simulink model "verify_ground_storage_U_tube_mdl"  (R2016b)
settings: Solver=ode45  StartTime=0  StopTime=2*3600  MaxStep=100  RelTol=1e-3  EnableMultiTasking=on
libraries: carnot x3, simulink x1
settings Model: Creator=drhf  LastModifiedBy=User
settings DataIOCC: SaveFormat=Array  SignalLoggingSaveFormat=ModelDataLogs
settings OptimizationCC: ExpressionDepthLimit=2147483647  LifeSpan=inf
settings DebuggingCC: UnderspecifiedInitializationDetection=Classic  MergeDetectMultiDrivingBlocksExec=none  SolverPrmCheckMsg=warning  FcnCallInpInsideContextMsg=warning  StateNameClashWarn=warning  SFUnexpectedBacktrackingDiag=warning  SFNoUnconditionalDefaultTransitionDiag=warning  SFExecutionAtInitializationDiag=none
settings HardwareCC: ProdBitPerPointer=32  ProdBitPerSizeT=32  ProdBitPerPtrDiffT=32  ProdLargestAtomicFloat=None  ProdIntDivRoundTo=Undefined  ProdEndianess=Unspecified  ProdWordSize=32  ProdHWDeviceType=32-bit Generic
settings ModelReferenceCC: PropagateSignalLabelsOutOfModel=off
settings GRTTargetCC: TargetLangStandard=C89/C90 (ANSI)  GeneratePreprocessorConditionals=Disable all  CombineOutputUpdateFcns=off  GRTInterface=on
settings ConfigComp: CovMetricSettings=dw  CovHtmlReporting=on  CovSaveCumulativeToWorkspaceVar=on  CovSaveSingleToWorkspaceVar=on  CovExternalEMLEnable=off

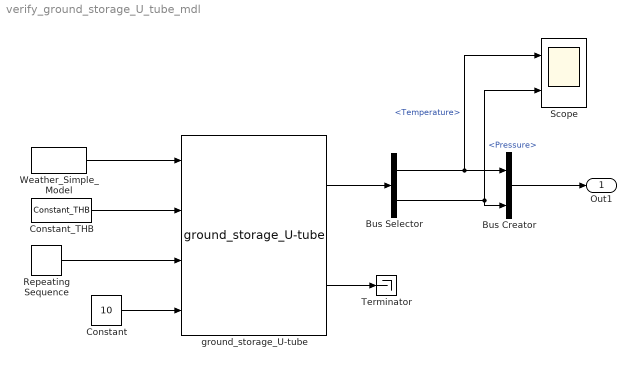
== system verify_ground_storage_U_tube_mdl ==
  Bus Creator : BusCreator  Inputs=2
  Bus Selector : BusSelector  OutputSignals=Temperature,Pressure
  Constant : Constant  Value=10
  Constant_THB : carnot/Source/Simple/Constant_THB  t=40  mdot=600/3600  p=1e5  mID=No Pressure Drop  fluid=Water  mix=0  mix2=0  mix3=0  dia=0.02  hgt=0
  Repeating Sequence : simulink/Sources/Repeating Sequence  rep_seq_t=[0 3600 2*3600]  rep_seq_y=[-5 10 -5]
  Scope : Scope  NumInputPorts=2
  Terminator : Terminator
  Weather_Simple_Model : carnot/Weather/Weather_Simple_Model  lat=60  Ibn=900  Idg=100  tamb=5  deltaTsky=-6  rh=50  precip="10e-3/24/3600           % 10 mm in 24 h"  cloud=0.125  p=1013e2  vw=1  wdir=270
  ground_storage_U-tube : carnot/New_Blocks/ground_storage_U-tube  ds=1  hs=1  dh=0.05  hh=1  ground=clay (humid)  borehole=clay (humid)  dp=0.02  kp=0.001  t0=10  rn=6  zn=6  mpts=3
  Out1 : Outport
  wires:
  Bus Creator/1 -> Out1/1
  Weather_Simple_Model/1 -> ground_storage_U-tube/1
  Constant_THB/1 -> ground_storage_U-tube/2
  Constant/1 -> ground_storage_U-tube/4
  Repeating Sequence/1 -> ground_storage_U-tube/3
  ground_storage_U-tube/1 -> Bus Selector/1
  Bus Selector/1 -> Scope/1, Bus Creator/1  "<Temperature>"
  Bus Selector/2 -> Scope/2, Bus Creator/2  "<Pressure>"
  ground_storage_U-tube/2 -> Terminator/1
